simulink model "slo_share_stream"  (R2015b)
settings: Solver=FixedStepDiscrete  SolverMode=SingleTasking  StartTime=0.0  StopTime=10  RelTol=1e-3
libraries: dspsrcs4 x1, simulink x1
CloseFcn:
  | rtwprivate ssgencode ModelCloseRequest Hysteresis_test1
settings Model: Creator=at-mt  LastModifiedBy=amatsumo
settings DataIOCC: SaveFormat=Array  SignalLoggingSaveFormat=ModelDataLogs  SaveOutput=off  SignalLogging=off  SaveTime=off
settings OptimizationCC: BlockReduction=off  ConditionallyExecuteInputs=off  DefaultParameterBehavior=Inlined  ExpressionDepthLimit=2147483647
settings DebuggingCC: AlgebraicLoopMsg=error  UnderspecifiedInitializationDetection=Classic  MergeDetectMultiDrivingBlocksExec=none  SolverPrmCheckMsg=warning  SingleTaskRateTransMsg=error  FcnCallInpInsideContextMsg=UseLocalSettings  StateNameClashWarn=warning
settings HardwareCC: ProdBitPerPointer=32  ProdLargestAtomicFloat=None  ProdIntDivRoundTo=Undefined  ProdEndianess=Unspecified  ProdWordSize=32  ProdHWDeviceType=ASIC/FPGA->ASIC/FPGA  ProdEqTarget=off
settings GRTTargetCC: GeneratePreprocessorConditionals=Disable all  CombineOutputUpdateFcns=off  GRTInterface=on
settings ConfigComp: CovModelRefEnable=Off  CovSFcnEnable=off

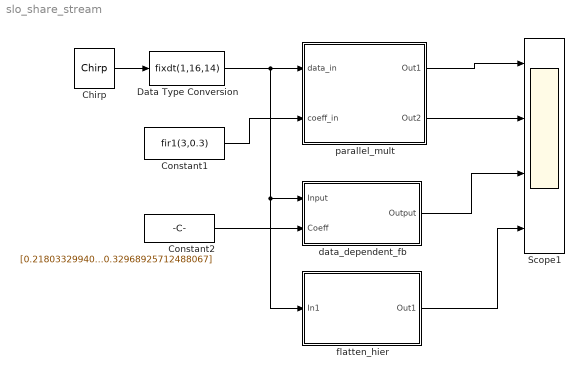
== system slo_share_stream ==
  Chirp : dspsrcs4/Chirp  sweep=Linear  mode=Unidirectional  f0=10  f1=500  t1=10  Tsweep=10  phase=0  Ts=1/1000  spf=1  datatype=Double  OutputFrames=on
  Constant1 : Constant  Value=fir1(3,0.3)  OutDataTypeStr=fixdt(1,16,14)  SampleTime=-1
  Constant2 : Constant  Value=[0.21803329940859612 1.9992290087844786 -0.35132832804499714 0.32968925712488067]  OutDataTypeStr=fixdt(1,16,14)  SampleTime=-1
  Data Type Conversion : DataTypeConversion  OutDataTypeStr=fixdt(1,16,14)
  Scope1 : Scope  NumInputPorts=4
  data_dependent_fb : Subsystem  Tag=FilterWizardSubSystem
      settings: ErrorFcn=dspFilterRealizedInBasicElemsAlgLoopErrFcnCallback
  flatten_hier : Subsystem
  parallel_mult : Subsystem
  wires:
  Chirp/1 -> Data Type Conversion/1
  Data Type Conversion/1 -> flatten_hier/1(In1), data_dependent_fb/1(Input), parallel_mult/1(data_in)
  Constant1/1 -> parallel_mult/2(coeff_in)
  parallel_mult/1(Out1) -> Scope1/1
  parallel_mult/2(Out2) -> Scope1/2
  data_dependent_fb/1(Output) -> Scope1/3
  Constant2/1 -> data_dependent_fb/2(Coeff)
  flatten_hier/1(Out1) -> Scope1/4

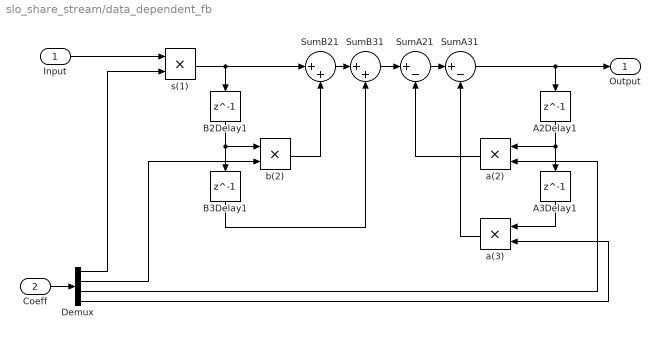
== system slo_share_stream/data_dependent_fb ==
  Input : Inport
  Coeff : Inport  Port=2
  A2Delay1 : Delay  DelayLength=1  InitialCondition=0
  A3Delay1 : Delay  DelayLength=1  InitialCondition=0
  B2Delay1 : Delay  DelayLength=1  InitialCondition=0
  B3Delay1 : Delay  DelayLength=1  InitialCondition=0
  Demux : Demux
  SumA21 : Sum  Inputs=|+-  RndMeth=Nearest  SaturateOnIntegerOverflow=on  OutDataTypeStr=Inherit: Same as first input
  SumA31 : Sum  Inputs=|+-  RndMeth=Nearest  SaturateOnIntegerOverflow=on  OutDataTypeStr=Inherit: Same as first input
  SumB21 : Sum  Inputs=|++  RndMeth=Nearest  SaturateOnIntegerOverflow=on  OutDataTypeStr=Inherit: Same as first input
  SumB31 : Sum  Inputs=|++  RndMeth=Nearest  SaturateOnIntegerOverflow=on  OutDataTypeStr=Inherit: Same as first input
  a(2) : Product  RndMeth=Nearest  OutDataTypeStr=Inherit: Same as first input
  a(3) : Product  RndMeth=Nearest  OutDataTypeStr=Inherit: Same as first input
  b(2) : Product  RndMeth=Nearest  OutDataTypeStr=Inherit: Same as first input
  s(1) : Product  RndMeth=Nearest  OutDataTypeStr=Inherit: Same as first input
  Output : Outport
  wires:
  Input/1 -> s(1)/1
  s(1)/1 -> SumB21/1, B2Delay1/1
  SumB21/1 -> SumB31/1
  SumB31/1 -> SumA21/1
  SumA21/1 -> SumA31/1
  SumA31/1 -> Output/1, A2Delay1/1
  B2Delay1/1 -> B3Delay1/1, b(2)/1
  b(2)/1 -> SumB21/2
  a(2)/1 -> SumA21/2
  A2Delay1/1 -> a(2)/1, A3Delay1/1
  B3Delay1/1 -> SumB31/2
  a(3)/1 -> SumA31/2
  A3Delay1/1 -> a(3)/1
  Coeff/1 -> Demux/1
  Demux/1 -> s(1)/2
  Demux/2 -> b(2)/2
  Demux/3 -> a(2)/2
  Demux/4 -> a(3)/2

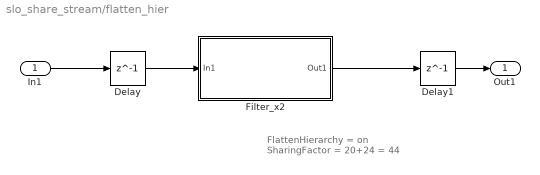
== system slo_share_stream/flatten_hier ==
  note: FlattenHierarchy = on
      | SharingFactor = 20+24 = 44
  In1 : Inport
  Delay : Delay  DelayLength=1
  Delay1 : Delay  DelayLength=1
  Filter_x2 : Subsystem
  Out1 : Outport
  wires:
  Filter_x2/1(Out1) -> Delay1/1
  Delay/1 -> Filter_x2/1(In1)
  Delay1/1 -> Out1/1
  In1/1 -> Delay/1

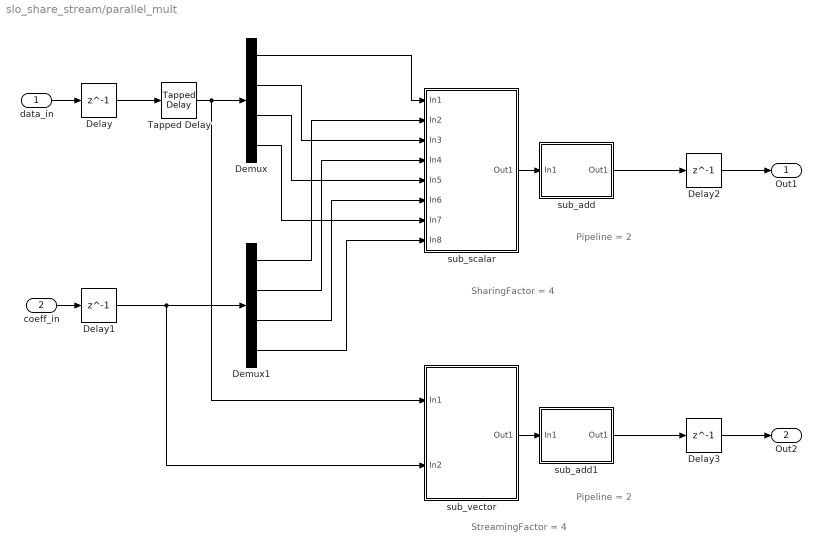
== system slo_share_stream/parallel_mult ==
  note: StreamingFactor = 4
  note: SharingFactor = 4
  note: Pipeline = 2
  note: Pipeline = 2
  data_in : Inport
  coeff_in : Inport  Port=2
  Delay{,1..3} (4 alike) : Delay  DelayLength=1
  Demux : Demux
  Demux1 : Demux
  Tapped Delay : simulink/Discrete/Tapped Delay  vinit=0.0  samptime=-1  NumDelays=3  DelayOrder=Oldest  includeCurrent=on
  sub_add : Subsystem
  sub_add1 : Subsystem
  sub_scalar : Subsystem
  sub_vector : Subsystem
  Out1 : Outport
  Out2 : Outport  Port=2
  wires:
  Delay/1 -> Tapped Delay/1
  coeff_in/1 -> Delay1/1
  Delay2/1 -> Out1/1
  data_in/1 -> Delay/1
  Tapped Delay/1 -> Demux/1, sub_vector/1(In1)
  Delay1/1 -> Demux1/1, sub_vector/2(In2)
  Demux/1 -> sub_scalar/1(In1)
  Demux/2 -> sub_scalar/3(In3)
  Demux/3 -> sub_scalar/5(In5)
  Demux/4 -> sub_scalar/7(In7)
  Demux1/1 -> sub_scalar/2(In2)
  Demux1/2 -> sub_scalar/4(In4)
  Demux1/3 -> sub_scalar/6(In6)
  Demux1/4 -> sub_scalar/8(In8)
  sub_scalar/1(Out1) -> sub_add/1(In1)
  sub_add/1(Out1) -> Delay2/1
  Delay3/1 -> Out2/1
  sub_add1/1(Out1) -> Delay3/1
  sub_vector/1(Out1) -> sub_add1/1(In1)

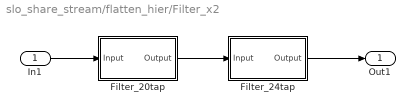
== system slo_share_stream/flatten_hier/Filter_x2 ==
  In1 : Inport
  Filter_20tap : Subsystem  Tag=FilterWizardSubSystem
      settings: ErrorFcn=dspFilterRealizedInBasicElemsAlgLoopErrFcnCallback
  Filter_24tap : Subsystem  Tag=FilterWizardSubSystem
      settings: ErrorFcn=dspFilterRealizedInBasicElemsAlgLoopErrFcnCallback
  Out1 : Outport
  wires:
  In1/1 -> Filter_20tap/1(Input)
  Filter_20tap/1(Output) -> Filter_24tap/1(Input)
  Filter_24tap/1(Output) -> Out1/1

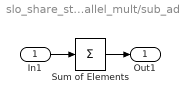
== system slo_share_stream/parallel_mult/sub_add ==
  In1 : Inport
  Sum of Elements : Sum  Inputs=+
  Out1 : Outport
  wires:
  In1/1 -> Sum of Elements/1
  Sum of Elements/1 -> Out1/1

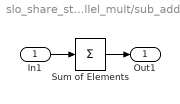
== system slo_share_stream/parallel_mult/sub_add1 ==
  In1 : Inport
  Sum of Elements : Sum  Inputs=+
  Out1 : Outport
  wires:
  Sum of Elements/1 -> Out1/1
  In1/1 -> Sum of Elements/1

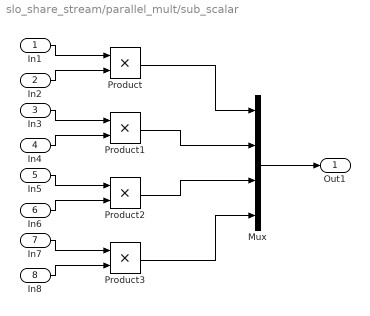
== system slo_share_stream/parallel_mult/sub_scalar ==
  In1 : Inport
  In2 : Inport  Port=2
  In3 : Inport  Port=3
  In4 : Inport  Port=4
  In5 : Inport  Port=5
  In6 : Inport  Port=6
  In7 : Inport  Port=7
  In8 : Inport  Port=8
  Mux : Mux
  Product{,1..3} (4 alike) : Product  RndMeth=Zero
  Out1 : Outport
  wires:
  In1/1 -> Product/1
  In2/1 -> Product/2
  In3/1 -> Product1/1
  In4/1 -> Product1/2
  Mux/1 -> Out1/1
  In5/1 -> Product2/1
  In6/1 -> Product2/2
  In7/1 -> Product3/1
  In8/1 -> Product3/2
  Product/1 -> Mux/1
  Product1/1 -> Mux/2
  Product2/1 -> Mux/3
  Product3/1 -> Mux/4

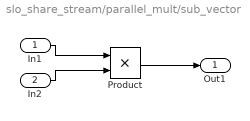
== system slo_share_stream/parallel_mult/sub_vector ==
  In1 : Inport
  In2 : Inport  Port=2
  Product : Product  RndMeth=Zero
  Out1 : Outport
  wires:
  In2/1 -> Product/2
  In1/1 -> Product/1
  Product/1 -> Out1/1

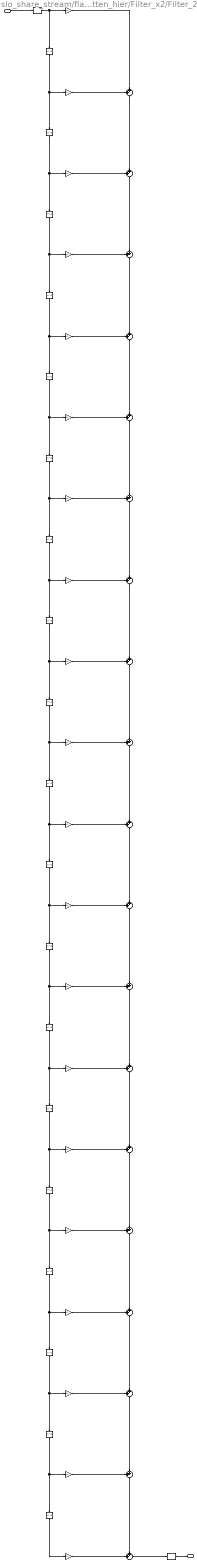
== system slo_share_stream/flatten_hier/Filter_x2/Filter_20tap ==
  Input : Inport
  BodyDelay{2..20} (19 alike) : Delay  DelayLength=1  InitialCondition=0  InputProcessing=Columns as channels (frame based)
  BodyLSum{2..20} (19 alike) : Sum  Inputs=++|  AccumDataTypeStr=fixdt(1,32,29)  OutDataTypeStr=fixdt(1,32,29)  RndMeth=Convergent
  ConvertIn : DataTypeConversion  OutDataTypeStr=fixdt(1,16,14)  RndMeth=Nearest  SaturateOnIntegerOverflow=on
  ConvertOut : DataTypeConversion  OutDataTypeStr=fixdt(1,32,29)  RndMeth=Convergent
  b(1) : Gain  Gain=0.0065785208536696949  ParamDataTypeStr=fixdt(1,16,15)  OutDataTypeStr=fixdt(1,31,29)  RndMeth=Convergent
  b(10) : Gain  Gain=0.56267500277478411  ParamDataTypeStr=fixdt(1,16,15)  OutDataTypeStr=fixdt(1,31,29)  RndMeth=Convergent
  b(11) : Gain  Gain=0.56267500277478411  ParamDataTypeStr=fixdt(1,16,15)  OutDataTypeStr=fixdt(1,31,29)  RndMeth=Convergent
  b(12) : Gain  Gain=-0.026694515910884429  ParamDataTypeStr=fixdt(1,16,15)  OutDataTypeStr=fixdt(1,31,29)  RndMeth=Convergent
  b(13) : Gain  Gain=-0.086100806895851215  ParamDataTypeStr=fixdt(1,16,15)  OutDataTypeStr=fixdt(1,31,29)  RndMeth=Convergent
  b(14) : Gain  Gain=0.074464270767581109  ParamDataTypeStr=fixdt(1,16,15)  OutDataTypeStr=fixdt(1,31,29)  RndMeth=Convergent
  b(15) : Gain  Gain=-0.019747599656098552  ParamDataTypeStr=fixdt(1,16,15)  OutDataTypeStr=fixdt(1,31,29)  RndMeth=Convergent
  b(16) : Gain  Gain=-0.020323357641311962  ParamDataTypeStr=fixdt(1,16,15)  OutDataTypeStr=fixdt(1,31,29)  RndMeth=Convergent
  b(17) : Gain  Gain=0.025637579992376872  ParamDataTypeStr=fixdt(1,16,15)  OutDataTypeStr=fixdt(1,31,29)  RndMeth=Convergent
  b(18) : Gain  Gain=-0.0099032805450486195  ParamDataTypeStr=fixdt(1,16,15)  OutDataTypeStr=fixdt(1,31,29)  RndMeth=Convergent
  b(19) : Gain  Gain=-0.0041930945382730499  ParamDataTypeStr=fixdt(1,16,15)  OutDataTypeStr=fixdt(1,31,29)  RndMeth=Convergent
  b(2) : Gain  Gain=-0.0041930945382730499  ParamDataTypeStr=fixdt(1,16,15)  OutDataTypeStr=fixdt(1,31,29)  RndMeth=Convergent
  b(20) : Gain  Gain=0.0065785208536696949  ParamDataTypeStr=fixdt(1,16,15)  OutDataTypeStr=fixdt(1,31,29)  RndMeth=Convergent
  b(3) : Gain  Gain=-0.0099032805450486195  ParamDataTypeStr=fixdt(1,16,15)  OutDataTypeStr=fixdt(1,31,29)  RndMeth=Convergent
  b(4) : Gain  Gain=0.025637579992376872  ParamDataTypeStr=fixdt(1,16,15)  OutDataTypeStr=fixdt(1,31,29)  RndMeth=Convergent
  b(5) : Gain  Gain=-0.020323357641311962  ParamDataTypeStr=fixdt(1,16,15)  OutDataTypeStr=fixdt(1,31,29)  RndMeth=Convergent
  b(6) : Gain  Gain=-0.019747599656098552  ParamDataTypeStr=fixdt(1,16,15)  OutDataTypeStr=fixdt(1,31,29)  RndMeth=Convergent
  b(7) : Gain  Gain=0.074464270767581109  ParamDataTypeStr=fixdt(1,16,15)  OutDataTypeStr=fixdt(1,31,29)  RndMeth=Convergent
  b(8) : Gain  Gain=-0.086100806895851215  ParamDataTypeStr=fixdt(1,16,15)  OutDataTypeStr=fixdt(1,31,29)  RndMeth=Convergent
  b(9) : Gain  Gain=-0.026694515910884429  ParamDataTypeStr=fixdt(1,16,15)  OutDataTypeStr=fixdt(1,31,29)  RndMeth=Convergent
  Output : Outport
  wires:
  ConvertOut/1 -> Output/1
  BodyLSum20/1 -> ConvertOut/1
  b(20)/1 -> BodyLSum20/2
  BodyDelay20/1 -> b(20)/1
  BodyLSum19/1 -> BodyLSum20/1
  b(19)/1 -> BodyLSum19/1
  BodyDelay19/1 -> BodyDelay20/1, b(19)/1
  BodyLSum18/1 -> BodyLSum19/2
  b(18)/1 -> BodyLSum18/1
  BodyDelay18/1 -> BodyDelay19/1, b(18)/1
  BodyLSum17/1 -> BodyLSum18/2
  b(17)/1 -> BodyLSum17/1
  BodyDelay17/1 -> BodyDelay18/1, b(17)/1
  BodyLSum16/1 -> BodyLSum17/2
  b(16)/1 -> BodyLSum16/1
  BodyDelay16/1 -> BodyDelay17/1, b(16)/1
  BodyLSum15/1 -> BodyLSum16/2
  b(15)/1 -> BodyLSum15/1
  BodyDelay15/1 -> BodyDelay16/1, b(15)/1
  BodyLSum14/1 -> BodyLSum15/2
  b(14)/1 -> BodyLSum14/1
  BodyDelay14/1 -> BodyDelay15/1, b(14)/1
  BodyLSum13/1 -> BodyLSum14/2
  b(13)/1 -> BodyLSum13/1
  BodyDelay13/1 -> BodyDelay14/1, b(13)/1
  BodyLSum12/1 -> BodyLSum13/2
  b(12)/1 -> BodyLSum12/1
  BodyDelay12/1 -> BodyDelay13/1, b(12)/1
  BodyLSum11/1 -> BodyLSum12/2
  b(11)/1 -> BodyLSum11/1
  BodyDelay11/1 -> BodyDelay12/1, b(11)/1
  BodyLSum10/1 -> BodyLSum11/2
  b(10)/1 -> BodyLSum10/1
  BodyDelay10/1 -> BodyDelay11/1, b(10)/1
  BodyLSum9/1 -> BodyLSum10/2
  b(9)/1 -> BodyLSum9/1
  BodyDelay9/1 -> BodyDelay10/1, b(9)/1
  BodyLSum8/1 -> BodyLSum9/2
  b(8)/1 -> BodyLSum8/1
  BodyDelay8/1 -> BodyDelay9/1, b(8)/1
  BodyLSum7/1 -> BodyLSum8/2
  b(7)/1 -> BodyLSum7/1
  BodyDelay7/1 -> BodyDelay8/1, b(7)/1
  BodyLSum6/1 -> BodyLSum7/2
  b(6)/1 -> BodyLSum6/1
  BodyDelay6/1 -> BodyDelay7/1, b(6)/1
  BodyLSum5/1 -> BodyLSum6/2
  b(5)/1 -> BodyLSum5/1
  BodyDelay5/1 -> BodyDelay6/1, b(5)/1
  BodyLSum4/1 -> BodyLSum5/2
  b(4)/1 -> BodyLSum4/1
  BodyDelay4/1 -> BodyDelay5/1, b(4)/1
  BodyLSum3/1 -> BodyLSum4/2
  b(3)/1 -> BodyLSum3/1
  BodyDelay3/1 -> BodyDelay4/1, b(3)/1
  BodyLSum2/1 -> BodyLSum3/2
  b(2)/1 -> BodyLSum2/1
  BodyDelay2/1 -> BodyDelay3/1, b(2)/1
  ConvertIn/1 -> BodyDelay2/1, b(1)/1
  b(1)/1 -> BodyLSum2/2
  Input/1 -> ConvertIn/1

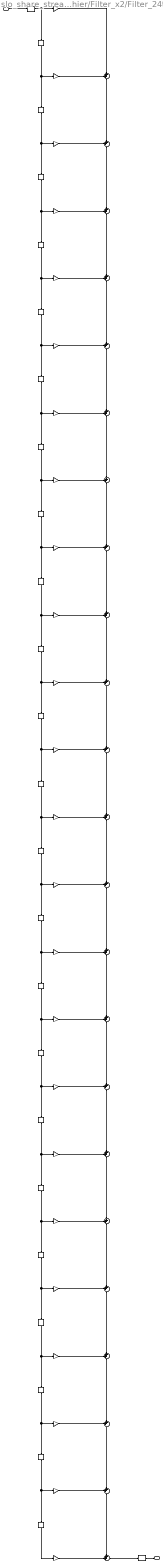
== system slo_share_stream/flatten_hier/Filter_x2/Filter_24tap ==
  Input : Inport
  BodyDelay{2..24} (23 alike) : Delay  DelayLength=1  InitialCondition=0  InputProcessing=Columns as channels (frame based)
  BodyLSum{2..24} (23 alike) : Sum  Inputs=++|  AccumDataTypeStr=fixdt(1,32,29)  OutDataTypeStr=fixdt(1,32,29)  RndMeth=Convergent
  ConvertIn : DataTypeConversion  OutDataTypeStr=fixdt(1,16,14)  RndMeth=Nearest  SaturateOnIntegerOverflow=on
  ConvertOut : DataTypeConversion  OutDataTypeStr=fixdt(1,32,29)  RndMeth=Convergent
  b(1) : Gain  Gain=0.0018103514622790915  ParamDataTypeStr=fixdt(1,16,15)  OutDataTypeStr=fixdt(1,31,29)  RndMeth=Convergent
  b(10) : Gain  Gain=0.079943707372564038  ParamDataTypeStr=fixdt(1,16,15)  OutDataTypeStr=fixdt(1,31,29)  RndMeth=Convergent
  b(11) : Gain  Gain=-0.037485856914524718  ParamDataTypeStr=fixdt(1,16,15)  OutDataTypeStr=fixdt(1,31,29)  RndMeth=Convergent
  b(12) : Gain  Gain=-0.5679645609678502  ParamDataTypeStr=fixdt(1,16,15)  OutDataTypeStr=fixdt(1,31,29)  RndMeth=Convergent
  b(13) : Gain  Gain=0.5679645609678502  ParamDataTypeStr=fixdt(1,16,15)  OutDataTypeStr=fixdt(1,31,29)  RndMeth=Convergent
  b(14) : Gain  Gain=0.037485856914524718  ParamDataTypeStr=fixdt(1,16,15)  OutDataTypeStr=fixdt(1,31,29)  RndMeth=Convergent
  b(15) : Gain  Gain=-0.079943707372564038  ParamDataTypeStr=fixdt(1,16,15)  OutDataTypeStr=fixdt(1,31,29)  RndMeth=Convergent
  b(16) : Gain  Gain=-0.078165912358661299  ParamDataTypeStr=fixdt(1,16,15)  OutDataTypeStr=fixdt(1,31,29)  RndMeth=Convergent
  b(17) : Gain  Gain=-0.028992378701570964  ParamDataTypeStr=fixdt(1,16,15)  OutDataTypeStr=fixdt(1,31,29)  RndMeth=Convergent
  b(18) : Gain  Gain=0.014408312807099323  ParamDataTypeStr=fixdt(1,16,15)  OutDataTypeStr=fixdt(1,31,29)  RndMeth=Convergent
  b(19) : Gain  Gain=0.027651241372913749  ParamDataTypeStr=fixdt(1,16,15)  OutDataTypeStr=fixdt(1,31,29)  RndMeth=Convergent
  b(2) : Gain  Gain=0.0059988467486783506  ParamDataTypeStr=fixdt(1,16,15)  OutDataTypeStr=fixdt(1,31,29)  RndMeth=Convergent
  b(20) : Gain  Gain=0.016573395978042922  ParamDataTypeStr=fixdt(1,16,15)  OutDataTypeStr=fixdt(1,31,29)  RndMeth=Convergent
  b(21) : Gain  Gain=0.00041059803043431921  ParamDataTypeStr=fixdt(1,16,15)  OutDataTypeStr=fixdt(1,31,29)  RndMeth=Convergent
  b(22) : Gain  Gain=-0.0073601585678137972  ParamDataTypeStr=fixdt(1,16,15)  OutDataTypeStr=fixdt(1,31,29)  RndMeth=Convergent
  b(23) : Gain  Gain=-0.0059988467486783506  ParamDataTypeStr=fixdt(1,16,15)  OutDataTypeStr=fixdt(1,31,29)  RndMeth=Convergent
  b(24) : Gain  Gain=-0.0018103514622790915  ParamDataTypeStr=fixdt(1,16,15)  OutDataTypeStr=fixdt(1,31,29)  RndMeth=Convergent
  b(3) : Gain  Gain=0.0073601585678137972  ParamDataTypeStr=fixdt(1,16,15)  OutDataTypeStr=fixdt(1,31,29)  RndMeth=Convergent
  b(4) : Gain  Gain=-0.00041059803043431921  ParamDataTypeStr=fixdt(1,16,15)  OutDataTypeStr=fixdt(1,31,29)  RndMeth=Convergent
  b(5) : Gain  Gain=-0.016573395978042922  ParamDataTypeStr=fixdt(1,16,15)  OutDataTypeStr=fixdt(1,31,29)  RndMeth=Convergent
  b(6) : Gain  Gain=-0.027651241372913749  ParamDataTypeStr=fixdt(1,16,15)  OutDataTypeStr=fixdt(1,31,29)  RndMeth=Convergent
  b(7) : Gain  Gain=-0.014408312807099323  ParamDataTypeStr=fixdt(1,16,15)  OutDataTypeStr=fixdt(1,31,29)  RndMeth=Convergent
  b(8) : Gain  Gain=0.028992378701570964  ParamDataTypeStr=fixdt(1,16,15)  OutDataTypeStr=fixdt(1,31,29)  RndMeth=Convergent
  b(9) : Gain  Gain=0.078165912358661299  ParamDataTypeStr=fixdt(1,16,15)  OutDataTypeStr=fixdt(1,31,29)  RndMeth=Convergent
  Output : Outport
  wires:
  ConvertOut/1 -> Output/1
  BodyLSum24/1 -> ConvertOut/1
  b(24)/1 -> BodyLSum24/2
  BodyDelay24/1 -> b(24)/1
  BodyLSum23/1 -> BodyLSum24/1
  b(23)/1 -> BodyLSum23/1
  BodyDelay23/1 -> BodyDelay24/1, b(23)/1
  BodyLSum22/1 -> BodyLSum23/2
  b(22)/1 -> BodyLSum22/1
  BodyDelay22/1 -> BodyDelay23/1, b(22)/1
  BodyLSum21/1 -> BodyLSum22/2
  b(21)/1 -> BodyLSum21/1
  BodyDelay21/1 -> BodyDelay22/1, b(21)/1
  BodyLSum20/1 -> BodyLSum21/2
  b(20)/1 -> BodyLSum20/1
  BodyDelay20/1 -> BodyDelay21/1, b(20)/1
  BodyLSum19/1 -> BodyLSum20/2
  b(19)/1 -> BodyLSum19/1
  BodyDelay19/1 -> BodyDelay20/1, b(19)/1
  BodyLSum18/1 -> BodyLSum19/2
  b(18)/1 -> BodyLSum18/1
  BodyDelay18/1 -> BodyDelay19/1, b(18)/1
  BodyLSum17/1 -> BodyLSum18/2
  b(17)/1 -> BodyLSum17/1
  BodyDelay17/1 -> BodyDelay18/1, b(17)/1
  BodyLSum16/1 -> BodyLSum17/2
  b(16)/1 -> BodyLSum16/1
  BodyDelay16/1 -> BodyDelay17/1, b(16)/1
  BodyLSum15/1 -> BodyLSum16/2
  b(15)/1 -> BodyLSum15/1
  BodyDelay15/1 -> BodyDelay16/1, b(15)/1
  BodyLSum14/1 -> BodyLSum15/2
  b(14)/1 -> BodyLSum14/1
  BodyDelay14/1 -> BodyDelay15/1, b(14)/1
  BodyLSum13/1 -> BodyLSum14/2
  b(13)/1 -> BodyLSum13/1
  BodyDelay13/1 -> BodyDelay14/1, b(13)/1
  BodyLSum12/1 -> BodyLSum13/2
  b(12)/1 -> BodyLSum12/1
  BodyDelay12/1 -> BodyDelay13/1, b(12)/1
  BodyLSum11/1 -> BodyLSum12/2
  b(11)/1 -> BodyLSum11/1
  BodyDelay11/1 -> BodyDelay12/1, b(11)/1
  BodyLSum10/1 -> BodyLSum11/2
  b(10)/1 -> BodyLSum10/1
  BodyDelay10/1 -> BodyDelay11/1, b(10)/1
  BodyLSum9/1 -> BodyLSum10/2
  b(9)/1 -> BodyLSum9/1
  BodyDelay9/1 -> BodyDelay10/1, b(9)/1
  BodyLSum8/1 -> BodyLSum9/2
  b(8)/1 -> BodyLSum8/1
  BodyDelay8/1 -> BodyDelay9/1, b(8)/1
  BodyLSum7/1 -> BodyLSum8/2
  b(7)/1 -> BodyLSum7/1
  BodyDelay7/1 -> BodyDelay8/1, b(7)/1
  BodyLSum6/1 -> BodyLSum7/2
  b(6)/1 -> BodyLSum6/1
  BodyDelay6/1 -> BodyDelay7/1, b(6)/1
  BodyLSum5/1 -> BodyLSum6/2
  b(5)/1 -> BodyLSum5/1
  BodyDelay5/1 -> BodyDelay6/1, b(5)/1
  BodyLSum4/1 -> BodyLSum5/2
  b(4)/1 -> BodyLSum4/1
  BodyDelay4/1 -> BodyDelay5/1, b(4)/1
  BodyLSum3/1 -> BodyLSum4/2
  b(3)/1 -> BodyLSum3/1
  BodyDelay3/1 -> BodyDelay4/1, b(3)/1
  BodyLSum2/1 -> BodyLSum3/2
  b(2)/1 -> BodyLSum2/1
  BodyDelay2/1 -> BodyDelay3/1, b(2)/1
  ConvertIn/1 -> BodyDelay2/1, b(1)/1
  b(1)/1 -> BodyLSum2/2
  Input/1 -> ConvertIn/1
